simulink model "NoC_4x4"  (R2015a)
settings: Solver=ode45  StartTime=0.0  StopTime=3000  FixedStep=1  RelTol=1e-3
undefined symbols (not defined in the file or in its folder): des, SELECT, T
libraries: simulink x16
(part 6 of 6)

== matlab function NoC_4x4/Router33/Attribute Function/MATLAB Function ==
  data: DST input; out_RT output; ME input
  events: trigger input FUNCTION_CALL_EVENT
function out_RT  = fcn(DST,ME)
%FCN    Access and modify attributes with MATLAB 
% 
% Input arguments must match the attribute names.
% Output arguments must be out_<AttributeName>,
% e.g., out_ServiceTime where ServiceTime is the attribute name.
% 
% The output attribute will be created if it is not present.
%

yi = floor(ME/4)+1;
xi = mod(ME,4);

if (xi==0),
    xi = 4;
    yi = yi - 1;
end

y = floor(DST/4)+1;
x = mod(DST,4);

if (x==0),
   x = 4;
    y = y - 1;
end

if x~=xi,
    if (x<xi),
        out_RT = 2;
    else 
        out_RT = 3;
    end
elseif y~=yi,
    if (y<yi),
        out_RT = 1;
    else
        out_RT = 4;
    end
else
    out_RT = 5;
end
